simulink model "simulink4"  (R2017a)
settings: Solver=VariableStepAuto  StartTime=0.0  StopTime=45  RelTol=1e-3
libraries: cstblocks x2
settings Model: Creator=Night_Fury  LastModifiedBy=Havoc

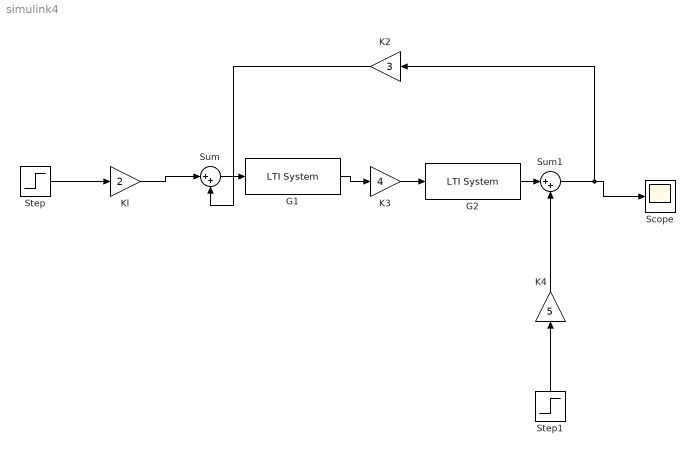
== system simulink4 ==
  "G1 " : cstblocks/LTI System  sys=tf([1],[1 1])  IC=[]
  G2 : cstblocks/LTI System  sys=tf([1],[1 1 8])  IC=[]
  K2 : Gain  Gain=3
  K3 : Gain  Gain=4
  K4 : Gain  Gain=5
  Kl : Gain  Gain=2
  Scope : Scope
  Step : Step  SampleTime=0
  Step1 : Step  SampleTime=0
  Sum : Sum  Inputs=|++
  Sum1 : Sum  Inputs=|++
  wires:
  K3/1 -> G2/1
  Step/1 -> Kl/1
  Kl/1 -> Sum/1
  Sum/1 -> "G1 "/1
  "G1 "/1 -> K3/1
  G2/1 -> Sum1/1
  Sum1/1 -> K2/1, Scope/1
  Step1/1 -> K4/1
  K4/1 -> Sum1/2
  K2/1 -> Sum/2
